simulink model "TLC"  (R2022b)
settings: configuration reference "ERT" (kept outside this file)
undefined symbols (not defined in the file): EGM, FID, IdcMin_P, kiIdcMax_P, kiIdcMin_P, kpIdcMax_P, kpIdcMin_P, OmMechnLimMin_P, pwrIdcMaxDev_P, pwrIdcMinDev_P, SC_fLoLim_C, SC_fUpLim_C, SC_PwrMax_P, SC_TrqMax_P, TQL, trqAddMax_P, trqAddMin_P, Ts_10ms
libraries: simulink x50, MathLib x8, DSMLib x2, slpidlib x1
(part 1 of 2)
settings Model: Creator=M00039784  LastModifiedBy=M00039784
settings ConfigSetRef: SourceName=ERT  SourceLocation=Base Workspace

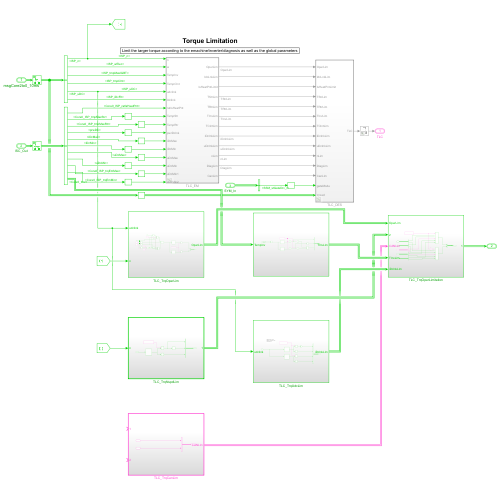
[thumbnail: Simulink's stored preview of the top-level diagram]
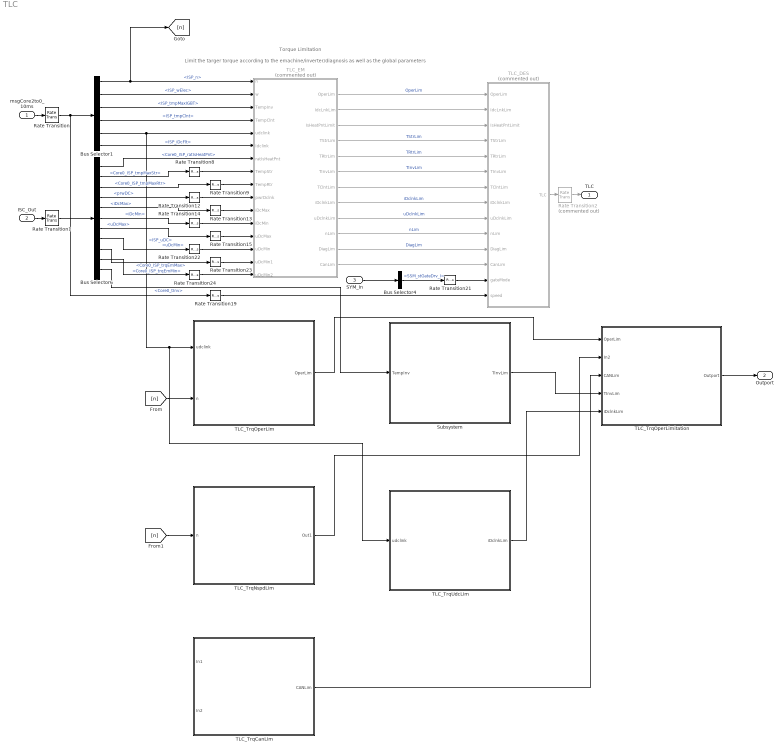
== system TLC ==
  note: Torque Limitation
  note: Limit the targer torque according to the emachine/inverter/diagnosis as well as the global parameters
  msgCore2to0_10ms : Inport  OutDataTypeStr=Bus: Sig10ms20ST
  ISC_Out : Inport  Port=2  OutDataTypeStr=Bus: Core0_ISP_Out
  SYM_In : Inport  Port=3  OutDataTypeStr=Bus: Core0_SSM_Out
  Bus Selector1 : BusSelector  OutputSignals=ISP_n,ISP_wElec,ISP_tmpMaxIGBT,ISP_tmpClnt,ISP_uDC,ISP_iDcFlt
  Bus Selector4 : BusSelector  OutputSignals=SSM_stGateDrv_I
  Bus Selector6 : BusSelector  OutputSignals=Core0_ISP_tmpOut.Core0_ISP_ratIsHeatPnt,Core0_ISP_tmpOut.Core0_ISP_tmpMaxStr,Core0_ISP_tmpOut.Core0_ISP_tmpMaxRtr,Core0_ISP_ComCmd.Core0_ISP_Dcx.prwDC,Core0_ISP_ComCmd.Core0_ISP_Dcx.iDcMax,Core0_ISP_ComCmd.Core0_ISP_Dcx.iDcMin,Core0_ISP_ComCmd.Core0_ISP_Dcx.uDcMax,Core0_ISP_ComCmd.Core0_ISP_Dcx.uDcMin,Core0_ISP_ComCmd.Core0_ISP_trqx.Core0_ISP_trqEmMax,Core0_ISP_ComCmd.Core0_ISP_trqx.Core0_ISP_trqEmMin,Core0_ISP_AnaOut.Core0_ISP_tInvx.Core0_tInv
  Rate Transition : RateTransition  OutPortSampleTime=Ts_10ms
  Rate Transition1 : RateTransition  OutPortSampleTime=Ts_10ms
  Rate Transition{8..9,12..15,19,22..24} (10 alike) : RateTransition
  Rate Transition2 : RateTransition  Commented=on  OutPortSampleTime=Ts_10ms
  Rate Transition21 : RateTransition  InitialCondition=EGM.Shortcircuit
  Subsystem : Subsystem
  TLC_DES : Subsystem  Commented=on  TreatAsAtomicUnit=on  SystemSampleTime=Ts_10ms
  TLC_EM : Subsystem  Commented=on  TreatAsAtomicUnit=on  SystemSampleTime=Ts_10ms
  TLC_TrqCanLim : Subsystem  TreatAsAtomicUnit=on
  TLC_TrqNspdLim : Subsystem  TreatAsAtomicUnit=on
  TLC_TrqOperLim : Subsystem
  TLC_TrqOperLimitation : Subsystem
  TLC_TrqUdcLim : Subsystem
  TLC : Outport  OutDataTypeStr=Bus: Core0_TLC_Out  VectorParamsAs1DForOutWhenUnconnected=off
  Outport : Outport  Port=2  OutDataTypeStr=Bus: Core0_TLC_TrqOut
  wires:
  TLC_EM/3(IsHeatPntLimit) -> TLC_DES/3(IsHeatPntLimit)
  Bus Selector6/1 -> TLC_EM/7(ratIsHeatPnt)  "<Core0_ISP_ratIsHeatPnt>"
  Bus Selector1/6 -> TLC_EM/6(Idclink)  "<ISP_iDcFlt>"
  TLC_EM/2(IdcLnkLim) -> TLC_DES/2(IdcLnkLim)
  Bus Selector1/5 -> TLC_TrqUdcLim/1(udclink), TLC_TrqOperLim/1(udclink), TLC_EM/5(udclink)  "<ISP_uDC>"
  Bus Selector6/10 -> Rate Transition24/1  "<Core0_ISP_trqEmMin>"
  Bus Selector1/3 -> TLC_EM/3(TempInv)  "<ISP_tmpMaxIGBT>"
  Bus Selector1/2 -> TLC_EM/2(w)  "<ISP_wElec>"
  SYM_In/1 -> Bus Selector4/1
  Bus Selector6/8 -> Rate Transition22/1  "<uDcMin>"
  TLC_EM/7(TClntLim) -> TLC_DES/7(TClntLim)
  Rate Transition19/1 -> TLC_DES/14(speed)
  Rate Transition24/1 -> TLC_EM/16(uDcMin2)
  Bus Selector6/7 -> Rate Transition15/1  "<uDcMax>"
  Bus Selector1/4 -> TLC_EM/4(TempClnt)  "<ISP_tmpClnt>"
  Bus Selector4/1 -> Rate Transition21/1  "<SSM_stGateDrv_I>"
  Bus Selector6/2 -> Rate Transition8/1  "<Core0_ISP_tmpMaxStr>"
  Rate Transition23/1 -> TLC_EM/15(uDcMin1)
  TLC_EM/8(iDclnkLim) -> TLC_DES/8(iDclnkLim)  "iDclnkLim"
  Rate Transition22/1 -> TLC_EM/14(uDcMin)
  Rate Transition12/1 -> TLC_EM/10(pwrDclnk)
  Rate Transition8/1 -> TLC_EM/8(TempStr)
  TLC_DES/1(TLC) -> Rate Transition2/1
  Rate Transition15/1 -> TLC_EM/13(uDcMax)
  Bus Selector6/4 -> Rate Transition12/1  "<prwDC>"
  Rate Transition14/1 -> TLC_EM/12(iDcMin)
  msgCore2to0_10ms/1 -> Rate Transition/1
  TLC_EM/5(TRtrLim) -> TLC_DES/5(TRtrLim)  "TRtrLim"
  Bus Selector6/3 -> Rate Transition9/1  "<Core0_ISP_tmpMaxRtr>"
  Bus Selector6/5 -> Rate Transition13/1  "<iDcMax>"
  TLC_EM/6(TInvLim) -> TLC_DES/6(TInvLim)  "TInvLim"
  ISC_Out/1 -> Rate Transition1/1
  TLC_EM/10(nLim) -> TLC_DES/10(nLim)  "nLim"
  TLC_EM/11(DiagLim) -> TLC_DES/11(DiagLim)  "DiagLim"
  Bus Selector1/1 -> [n], TLC_EM/1(n)  "<ISP_n>"
  TLC_EM/4(TStrLim) -> TLC_DES/4(TStrLim)  "TStrLim"
  TLC_EM/1(OperLim) -> TLC_DES/1(OperLim)  "OperLim"
  Bus Selector6/6 -> Rate Transition14/1  "<iDcMin>"
  TLC_EM/9(uDclnkLim) -> TLC_DES/9(uDclnkLim)  "uDclnkLim"
  Rate Transition21/1 -> TLC_DES/13(gateMode)
  Bus Selector6/9 -> Rate Transition23/1  "<Core0_ISP_trqEmMax>"
  TLC_EM/12(CanLim) -> TLC_DES/12(CanLim)
  Rate Transition9/1 -> TLC_EM/9(TempRtr)
  Rate Transition13/1 -> TLC_EM/11(iDcMax)
  Rate Transition/1 -> Rate Transition19/1, Bus Selector1/1
  Rate Transition1/1 -> Bus Selector6/1
  Rate Transition2/1 -> TLC/1
  [n] -> TLC_TrqOperLim/2(n)
  [n] -> TLC_TrqNspdLim/1(n)
  TLC_TrqOperLim/1(OperLim) -> TLC_TrqOperLimitation/1(OperLim)
  TLC_TrqNspdLim/1(Out1) -> TLC_TrqOperLimitation/2(In2)
  TLC_TrqCanLim/1(CANLim) -> TLC_TrqOperLimitation/3(CANLim)
  Subsystem/1(TInvLim) -> TLC_TrqOperLimitation/4(TInvLim)
  TLC_TrqUdcLim/1(iDclnkLim) -> TLC_TrqOperLimitation/5(iDclnkLim)
  TLC_TrqOperLimitation/1(Outport) -> Outport/1
  Bus Selector6/11 -> Subsystem/1(TempInv)  "<Core0_tInv>"

== system TLC/Subsystem ==
  TempInv : Inport
  Bus Creator : BusCreator  Inputs=3
  Bus Selector : BusSelector  OutputSignals=Core0_ISP_IGBTTemp1,Core0_ISP_IGBTTemp2
  GLB_TrqMax_P2 : Constant  Value=SC_TrqMax_P  OutDataTypeStr=single
  Logical Operator : Logic  Operator=OR  AllPortsSameDT=off  OutDataTypeStr=boolean
  Max : MinMax  Function=max  Inputs=2
  Product : Product
  Product1 : Product
  Relational Operator : RelationalOperator  OutDataTypeStr=boolean  RndMeth=Simplest  InputSameDT=off
  Relational Operator1 : RelationalOperator  OutDataTypeStr=boolean  RndMeth=Simplest  InputSameDT=off
  Unary Minus : UnaryMinus
  trqGenTInvLim_T : Lookup_n-D  NumberOfTableDimensions=1  DataSpecification=Lookup table object  LookupTableObject=trqGenTInvLim_T  BreakpointsForDimension1=[100 125 135]  BeginIndexSearchUsingPreviousIndexResult=on  Table=[1 0.8 0]  ExtrapMethod=Clip  UseLastTableValue=on  InternalRulePriority=Speed  OutDataTypeStr=Inherit: Inherit from 'Table data'  RndMeth=Simplest
  trqMotTInvLim_T : Lookup_n-D  NumberOfTableDimensions=1  DataSpecification=Lookup table object  LookupTableObject=trqMotTInvLim_T  BreakpointsForDimension1=[100 125 135]  BeginIndexSearchUsingPreviousIndexResult=on  Table=[1 0.8 0]  ExtrapMethod=Clip  UseLastTableValue=on  InternalRulePriority=Speed  OutDataTypeStr=Inherit: Inherit from 'Table data'  RndMeth=Simplest
  TInvLim : Outport  VectorParamsAs1DForOutWhenUnconnected=off
  wires:
  Logical Operator/1 -> Bus Creator/3  "bTrqTinvLimActv"
  trqGenTInvLim_T/1 -> Product1/2
  Relational Operator1/1 -> Logical Operator/2  "bTrqGenTInvLimActv"
  Bus Creator/1 -> TInvLim/1
  Relational Operator/1 -> Logical Operator/1  "bTrqMotTInvLimActv"
  GLB_TrqMax_P2/1 -> Relational Operator1/1, Relational Operator/1, Product1/1, Product/1
  trqMotTInvLim_T/1 -> Product/2
  Product1/1 -> Unary Minus/1, Relational Operator1/2
  Unary Minus/1 -> Bus Creator/2  "trqGenTInvLim"
  Max/1 -> trqGenTInvLim_T/1, trqMotTInvLim_T/1
  Product/1 -> Bus Creator/1, Relational Operator/2  "trqMotTInvLim"
  TempInv/1 -> Bus Selector/1
  Bus Selector/1 -> Max/1  "<Core0_ISP_IGBTTemp1>"
  Bus Selector/2 -> Max/2  "<Core0_ISP_IGBTTemp2>"

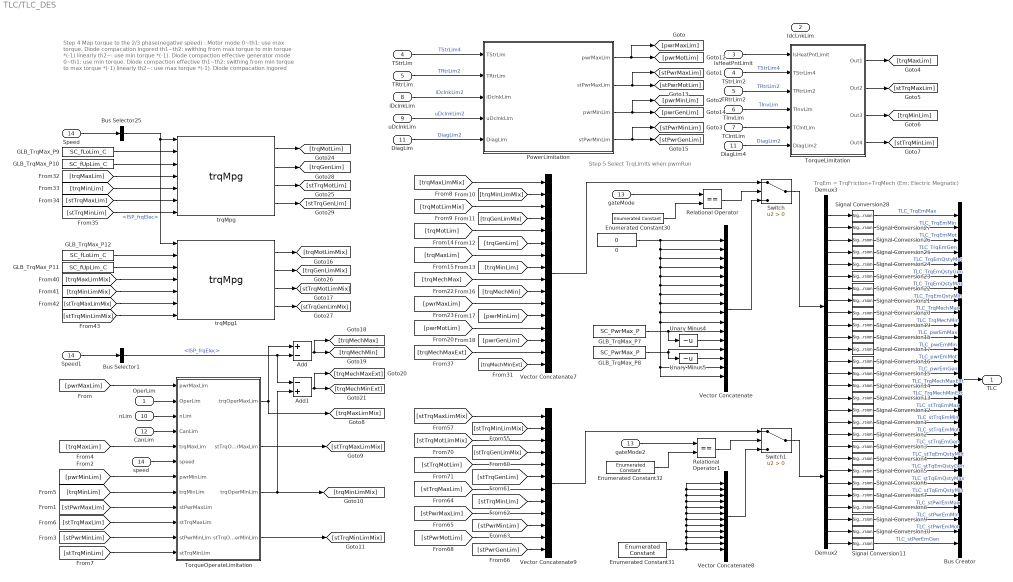
== system TLC/TLC_DES ==
  note: Step 4 Map torque to the 2/3 phase(negative speed) :
      | Motor mode
      | 0~th1: use max torque. Diode compacation ingored
      | th1~th2: swithing from max torque to min torque *(-1) linearly
      | th2~: use min torque *(-1). Diode compaction effective
      | generator mode
      | 0~th1: use min torque. Diode compaction effective
      | th1~th2: swithing from min torque to max torque *(-1) linearly
      | th2~: use max torque *(-1). Diode compacation ingored
  note: TrqEm = TrqFriction+TrqMech (Em: Electric Megnatic)
  note: Step 5 Select TrqLimits when pwmRun
  OperLim : Inport
  IdcLnkLim : Inport  Port=2
  IsHeatPntLimit : Inport  Port=3
  TStrLim : Inport  Port=4
  TRtrLim : Inport  Port=5
  TInvLim : Inport  Port=6
  TClntLim : Inport  Port=7
  iDclnkLim : Inport  Port=8
  uDclnkLim : Inport  Port=9
  nLim : Inport  Port=10
  DiagLim : Inport  Port=11
  CanLim : Inport  Port=12
  gateMode : Inport  Port=13
  speed : Inport  Port=14
  0 : Constant  Value=0  OutDataTypeStr=single
  Add : Sum  Inputs=+-
  Add1 : Sum  Inputs=-+
  Bus Creator : BusCreator  Inputs=28
  Bus Selector1 : BusSelector  OutputSignals=ISP_frqElec
  Bus Selector25 : BusSelector  OutputSignals=ISP_frqElec
  Demux2 : Demux  Outputs=12
  Demux3 : Demux  Outputs=16
  DiagLim4 : InportShadow  Port=11
  Enumerated Constant30 : simulink/Sources/Enumerated Constant  OutDataTypeStr=Enum: EGM  Value=EGM.PWMRun  SampleTime=inf
  Enumerated Constant31 : simulink/Sources/Enumerated Constant  OutDataTypeStr=Enum: TQL  Value=TQL.Inactive  SampleTime=inf
  Enumerated Constant32 : simulink/Sources/Enumerated Constant  OutDataTypeStr=Enum: EGM  Value=EGM.PWMRun  SampleTime=inf
  GLB_TrqMax_P10 : Constant  Value=SC_fUpLim_C  OutDataTypeStr=single
  GLB_TrqMax_P11 : Constant  Value=SC_fUpLim_C  OutDataTypeStr=single
  GLB_TrqMax_P12 : Constant  Value=SC_fLoLim_C  OutDataTypeStr=single
  GLB_TrqMax_P7 : Constant  Value=SC_PwrMax_P  OutDataTypeStr=single
  GLB_TrqMax_P8 : Constant  Value=SC_PwrMax_P  OutDataTypeStr=single
  GLB_TrqMax_P9 : Constant  Value=SC_fLoLim_C  OutDataTypeStr=single
  PowerLimitation : Subsystem
  Relational Operator : RelationalOperator  Operator===  OutDataTypeStr=boolean  RndMeth=Simplest  InputSameDT=off
  Relational Operator1 : RelationalOperator  Operator===  OutDataTypeStr=boolean  RndMeth=Simplest  InputSameDT=off
  Signal Conversion{1..28} (28 alike) : SignalConversion  OverrideOpt=off
  Speed : InportShadow  Port=14
  Speed1 : InportShadow  Port=14
  Switch : Switch  Criteria=u2 > Threshold  SaturateOnIntegerOverflow=off  InputSameDT=off
  Switch1 : Switch  Criteria=u2 > Threshold  SaturateOnIntegerOverflow=off  InputSameDT=off
  TRtrLim2 : InportShadow  Port=5
  TStrLim2 : InportShadow  Port=4
  TorqueLimitation : Subsystem
  TorqueOperateLimitation : Subsystem
  Unary Minus4 : UnaryMinus
  Unary Minus5 : UnaryMinus
  Vector Concatenate : Concatenate  NumInputs=16
  Vector Concatenate7 : Concatenate  NumInputs=16
  Vector Concatenate8 : Concatenate  NumInputs=12
  Vector Concatenate9 : Concatenate  NumInputs=12
  gateMode2 : InportShadow  Port=13
  trqMpg : MathLib/trqMpg  SystemSampleTime=-1  VariantActivationTime=update diagram  Latency=0  AutoFrameSizeCalculation=off
  trqMpg1 : MathLib/trqMpg  SystemSampleTime=-1  VariantActivationTime=update diagram  Latency=0  AutoFrameSizeCalculation=off
  TLC : Outport  VectorParamsAs1DForOutWhenUnconnected=off
  wires:
  Speed/1 -> Bus Selector25/1
  trqMpg/1 -> [trqMotLim]
  trqMpg/3 -> [stTrqMotLim]
  trqMpg/2 -> [trqGenLim]
  trqMpg/4 -> [stTrqGenLim]
  Bus Selector25/1 -> trqMpg1/1, trqMpg/1  "<ISP_frqElec>"
  trqMpg1/1 -> [trqMotLimMix]
  trqMpg1/3 -> [stTrqMotLimMix]
  trqMpg1/2 -> [trqGenLimMix]
  trqMpg1/4 -> [stTrqGenLimMix]
  TorqueOperateLimitation/1(trqOperMaxLim) -> [trqMaxLimMix], Add/1
  TorqueOperateLimitation/3(trqOperMinLim) -> Add1/2, [trqMinLimMix]
  Bus Selector1/1 -> Add1/1, Add/2  "<ISP_frqElec>"
  Add/1 -> [trqMechMax], [trqMechMin]
  Add1/1 -> [trqMechMaxExt], [trqMechMinExt]
  [stTrqMinLim] -> trqMpg/7
  [stTrqMaxLim] -> trqMpg/6
  [trqMinLim] -> trqMpg/5
  [trqMaxLim] -> trqMpg/4
  GLB_TrqMax_P9/1 -> trqMpg/2
  GLB_TrqMax_P10/1 -> trqMpg/3
  [stTrqMinLimMix] -> trqMpg1/7
  [stTrqMaxLimMix] -> trqMpg1/6
  [trqMinLimMix] -> trqMpg1/5
  [trqMaxLimMix] -> trqMpg1/4
  GLB_TrqMax_P12/1 -> trqMpg1/2
  GLB_TrqMax_P11/1 -> trqMpg1/3
  PowerLimitation/1(pwrMaxLim) -> [pwrMaxLim], [pwrMotLim]
  PowerLimitation/2(stPwrMaxLim) -> [stPwrMaxLim], [stPwrMotLim]
  PowerLimitation/3(pwrMinLim) -> [pwrMinLim], [pwrGenLim]
  PowerLimitation/4(stPwrMinLim) -> [stPwrMinLim], [stPwrGenLim]
  TStrLim/1 -> PowerLimitation/1(TStrLim)  "TStrLim4"
  TRtrLim/1 -> PowerLimitation/2(TRtrLim)  "TRtrLim2"
  iDclnkLim/1 -> PowerLimitation/3(iDclnkLim)  "iDclnkLim2"
  uDclnkLim/1 -> PowerLimitation/4(uDclnkLim)  "uDclnkLim2"
  DiagLim/1 -> PowerLimitation/5(DiagLim)  "DiagLim2"
  TStrLim2/1 -> TorqueLimitation/2(TStrLim4)  "TStrLim4"
  TRtrLim2/1 -> TorqueLimitation/3(TRtrLim2)  "TRtrLim2"
  TInvLim/1 -> TorqueLimitation/4(TInvLim)  "TInvLim"
  DiagLim4/1 -> TorqueLimitation/6(DiagLim2)  "DiagLim2"
  TorqueLimitation/1(Out1) -> [trqMaxLim]
  TorqueLimitation/2(Out2) -> [stTrqMaxLim]
  TorqueLimitation/3(Out3) -> [trqMinLim]
  TorqueLimitation/4(Out4) -> [stTrqMinLim]
  [pwrMaxLim] -> TorqueOperateLimitation/1(pwrMaxLim)
  OperLim/1 -> TorqueOperateLimitation/2(OperLim)
  nLim/1 -> TorqueOperateLimitation/3(nLim)
  CanLim/1 -> TorqueOperateLimitation/4(CanLim)
  [trqMaxLim] -> TorqueOperateLimitation/5(trqMaxLim)
  speed/1 -> TorqueOperateLimitation/6(speed)
  [pwrMinLim] -> TorqueOperateLimitation/7(pwrMinLim)
  [trqMinLim] -> TorqueOperateLimitation/8(trqMinLim)
  TorqueOperateLimitation/2(stTrqOperMaxLim) -> [stTrqMaxLimMix]
  TorqueOperateLimitation/4(stTrqOperMinLim) -> [stTrqMinLimMix]
  [stPwrMaxLim] -> TorqueOperateLimitation/9(stPwrMaxLim)
  [stTrqMaxLim] -> TorqueOperateLimitation/10(stTrqMaxLim)
  [stTrqMinLim] -> TorqueOperateLimitation/12(stTrqMinLim)
  [stPwrMinLim] -> TorqueOperateLimitation/11(stPwrMinLim)
  Enumerated Constant30/1 -> Relational Operator/2
  Relational Operator/1 -> Switch/2
  0/1 -> Vector Concatenate/2, Vector Concatenate/3, Vector Concatenate/4, Vector Concatenate/5, Vector Concatenate/6, Vector Concatenate/7, Vector Concatenate/8, Vector Concatenate/9, Vector Concatenate/10, Vector Concatenate/16, Vector Concatenate/15, Vector Concatenate/1
  GLB_TrqMax_P7/1 -> Vector Concatenate/11, Unary Minus4/1
  GLB_TrqMax_P8/1 -> Vector Concatenate/13, Unary Minus5/1
  Demux3/7 -> Signal Conversion22/1
  Demux3/6 -> Signal Conversion23/1
  Demux3/8 -> Signal Conversion21/1
  Demux3/5 -> Signal Conversion24/1
  Demux3/9 -> Signal Conversion20/1
  Demux3/4 -> Signal Conversion25/1
  Demux3/3 -> Signal Conversion26/1
  Demux3/10 -> Signal Conversion19/1
  Demux3/2 -> Signal Conversion27/1
  Demux3/11 -> Signal Conversion18/1
  Demux3/1 -> Signal Conversion28/1
  Demux3/12 -> Signal Conversion17/1
  Demux3/13 -> Signal Conversion16/1
  Demux3/14 -> Signal Conversion15/1
  Demux2/1 -> Signal Conversion12/1
  Demux2/2 -> Signal Conversion1/1
  Demux2/3 -> Signal Conversion2/1
  Demux2/4 -> Signal Conversion3/1
  Demux2/5 -> Signal Conversion4/1
  Demux2/6 -> Signal Conversion5/1
  Demux2/7 -> Signal Conversion6/1
  Demux2/8 -> Signal Conversion7/1
  Demux2/9 -> Signal Conversion8/1
  Demux2/10 -> Signal Conversion9/1
  Demux2/11 -> Signal Conversion10/1
  Demux2/12 -> Signal Conversion11/1
  Demux3/15 -> Signal Conversion14/1
  Demux3/16 -> Signal Conversion13/1
  [trqMotLimMix] -> Vector Concatenate7/3
  [trqMaxLimMix] -> Vector Concatenate7/1
  [trqMinLimMix] -> Vector Concatenate7/2
  Vector Concatenate7/1 -> Switch/1
  Vector Concatenate/1 -> Switch/3
  Switch/1 -> Demux3/1
  [trqGenLimMix] -> Vector Concatenate7/4
  [trqMaxLim] -> Vector Concatenate7/7
  [trqMotLim] -> Vector Concatenate7/5
  [trqGenLim] -> Vector Concatenate7/6
  [trqMinLim] -> Vector Concatenate7/8
  [pwrMaxLim] -> Vector Concatenate7/11
  [trqMechMax] -> Vector Concatenate7/9
  [pwrMotLim] -> Vector Concatenate7/13
  [trqMechMaxExt] -> Vector Concatenate7/15
  [trqMechMinExt] -> Vector Concatenate7/16
  [pwrGenLim] -> Vector Concatenate7/14
  [trqMechMin] -> Vector Concatenate7/10
  [pwrMinLim] -> Vector Concatenate7/12
  Bus Creator/1 -> TLC/1
  Unary Minus5/1 -> Vector Concatenate/14
  Unary Minus4/1 -> Vector Concatenate/12
  Enumerated Constant31/1 -> Vector Concatenate8/1, Vector Concatenate8/2, Vector Concatenate8/3, Vector Concatenate8/4, Vector Concatenate8/5, Vector Concatenate8/6, Vector Concatenate8/7, Vector Concatenate8/8, Vector Concatenate8/9, Vector Concatenate8/10, Vector Concatenate8/11, Vector Concatenate8/12
  Vector Concatenate9/1 -> Switch1/1
  [stPwrGenLim] -> Vector Concatenate9/12
  [stPwrMinLim] -> Vector Concatenate9/10
  [stTrqMinLim] -> Vector Concatenate9/8
  [stTrqGenLim] -> Vector Concatenate9/6
  [stTrqGenLimMix] -> Vector Concatenate9/4
  [stPwrMotLim] -> Vector Concatenate9/11
  [stTrqMinLimMix] -> Vector Concatenate9/2
  [stPwrMaxLim] -> Vector Concatenate9/9
  [stTrqMaxLim] -> Vector Concatenate9/7
  [stTrqMotLim] -> Vector Concatenate9/5
  [stTrqMotLimMix] -> Vector Concatenate9/3
  [stTrqMaxLimMix] -> Vector Concatenate9/1
  Enumerated Constant32/1 -> Relational Operator1/2
  Relational Operator1/1 -> Switch1/2
  Vector Concatenate8/1 -> Switch1/3
  Switch1/1 -> Demux2/1
  Signal Conversion1/1 -> Bus Creator/18  "TLC_stTrqEmMin"
  Signal Conversion2/1 -> Bus Creator/19  "TLC_stTrqEmMot"
  Signal Conversion3/1 -> Bus Creator/20  "TLC_stTrqEmGen"
  Signal Conversion4/1 -> Bus Creator/21  "TLC_stTqEmQstyMot"
  Signal Conversion5/1 -> Bus Creator/22  "TLC_stTqEmQstyGen"
  Signal Conversion6/1 -> Bus Creator/23  "TLC_stTqEmQstyMax"
  Signal Conversion7/1 -> Bus Creator/24  "TLC_stTqEmQstyMin"
  Signal Conversion8/1 -> Bus Creator/25  "TLC_stPwrEmMax"
  Signal Conversion9/1 -> Bus Creator/26  "TLC_stPwrEmMin"
  Signal Conversion10/1 -> Bus Creator/27  "TLC_stPwrEmMot"
  Signal Conversion11/1 -> Bus Creator/28  "TLC_stPwrEmGen"
  Signal Conversion12/1 -> Bus Creator/17  "TLC_stTrqEmMax"
  Signal Conversion13/1 -> Bus Creator/16  "TLC_TrqMechMinExt"
  Signal Conversion14/1 -> Bus Creator/15  "TLC_TrqMechMaxExt"
  Signal Conversion15/1 -> Bus Creator/14  "TLC_pwrEmGen"
  Signal Conversion16/1 -> Bus Creator/13  "TLC_pwrEmMot"
  Signal Conversion17/1 -> Bus Creator/12  "TLC_pwrEmMin"
  Signal Conversion18/1 -> Bus Creator/11  "TLC_pwrEmMax"
  Signal Conversion19/1 -> Bus Creator/10  "TLC_TrqMechMin"
  Signal Conversion20/1 -> Bus Creator/9  "TLC_TrqMechMax"
  Signal Conversion21/1 -> Bus Creator/8  "TLC_TrqEmQstyMin"
  Signal Conversion22/1 -> Bus Creator/7  "TLC_TrqEmQstyMax"
  Signal Conversion23/1 -> Bus Creator/6  "TLC_TrqEmQstyGen"
  Signal Conversion24/1 -> Bus Creator/5  "TLC_TrqEmQstyMot"
  Signal Conversion25/1 -> Bus Creator/4  "TLC_TrqEmGen"
  Signal Conversion26/1 -> Bus Creator/3  "TLC_TrqEmMot"
  Signal Conversion27/1 -> Bus Creator/2  "TLC_TrqEmMin"
  Signal Conversion28/1 -> Bus Creator/1  "TLC_TrqEmMax"
  gateMode/1 -> Relational Operator/1
  gateMode2/1 -> Relational Operator1/1
  Speed1/1 -> Bus Selector1/1
  IsHeatPntLimit/1 -> TorqueLimitation/1(IsHeatPntLimit)
  TClntLim/1 -> TorqueLimitation/5(TClntLim)

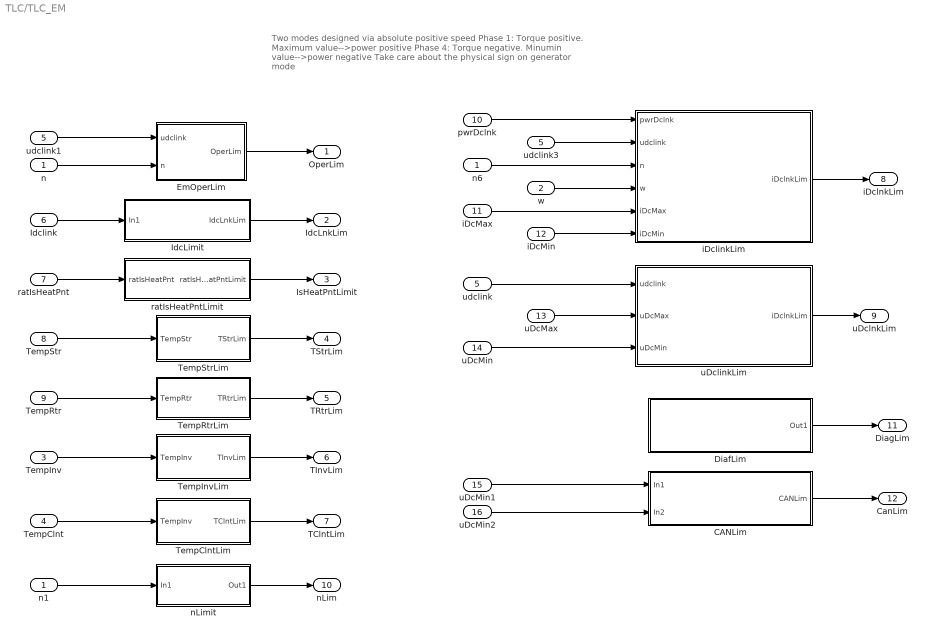
== system TLC/TLC_EM ==
  note: Two modes designed via absolute positive speed
      | Phase 1: Torque  positive. Maximum value-->power positive
      | Phase 4: Torque negative. Minumin value-->power negative
      | Take care about the physical sign on generator mode
  n : Inport
  w : Inport  Port=2
  TempInv : Inport  Port=3
  TempClnt : Inport  Port=4
  udclink : Inport  Port=5
  Idclink : Inport  Port=6
  ratIsHeatPnt : Inport  Port=7
  TempStr : Inport  Port=8
  TempRtr : Inport  Port=9
  pwrDclnk : Inport  Port=10
  iDcMax : Inport  Port=11
  iDcMin : Inport  Port=12
  uDcMax : Inport  Port=13
  uDcMin : Inport  Port=14
  uDcMin1 : Inport  Port=15
  uDcMin2 : Inport  Port=16
  CANLim : Subsystem  TreatAsAtomicUnit=on
  DiafLim : Subsystem  TreatAsAtomicUnit=on
  EmOperLim : Subsystem  TreatAsAtomicUnit=on
  IdcLimit : Subsystem  TreatAsAtomicUnit=on
  TempClntLim : Subsystem  TreatAsAtomicUnit=on
  TempInvLim : Subsystem  TreatAsAtomicUnit=on
  TempRtrLim : Subsystem  TreatAsAtomicUnit=on
  TempStrLim : Subsystem  TreatAsAtomicUnit=on
  iDclinkLim : Subsystem  TreatAsAtomicUnit=on
  n1 : InportShadow
  n6 : InportShadow
  nLimit : Subsystem  TreatAsAtomicUnit=on
  ratIsHeatPntLimit : Subsystem  TreatAsAtomicUnit=on
  uDclinkLim : Subsystem  TreatAsAtomicUnit=on
  udclink1 : InportShadow  Port=5
  udclink3 : InportShadow  Port=5
  OperLim : Outport  VectorParamsAs1DForOutWhenUnconnected=off
  IdcLnkLim : Outport  Port=2  VectorParamsAs1DForOutWhenUnconnected=off
  IsHeatPntLimit : Outport  Port=3  VectorParamsAs1DForOutWhenUnconnected=off
  TStrLim : Outport  Port=4  VectorParamsAs1DForOutWhenUnconnected=off
  TRtrLim : Outport  Port=5  VectorParamsAs1DForOutWhenUnconnected=off
  TInvLim : Outport  Port=6  VectorParamsAs1DForOutWhenUnconnected=off
  TClntLim : Outport  Port=7  VectorParamsAs1DForOutWhenUnconnected=off
  iDclnkLim : Outport  Port=8  VectorParamsAs1DForOutWhenUnconnected=off
  uDclnkLim : Outport  Port=9  VectorParamsAs1DForOutWhenUnconnected=off
  nLim : Outport  Port=10  VectorParamsAs1DForOutWhenUnconnected=off
  DiagLim : Outport  Port=11  VectorParamsAs1DForOutWhenUnconnected=off
  CanLim : Outport  Port=12  VectorParamsAs1DForOutWhenUnconnected=off
  wires:
  TempInvLim/1(TInvLim) -> TInvLim/1
  TempInv/1 -> TempInvLim/1(TempInv)
  udclink1/1 -> EmOperLim/1(udclink)
  n/1 -> EmOperLim/2(n)
  EmOperLim/1(OperLim) -> OperLim/1
  TempStr/1 -> TempStrLim/1(TempStr)
  TempStrLim/1(TStrLim) -> TStrLim/1
  TempRtr/1 -> TempRtrLim/1(TempRtr)
  TempRtrLim/1(TRtrLim) -> TRtrLim/1
  udclink3/1 -> iDclinkLim/2(udclink)
  n6/1 -> iDclinkLim/3(n)
  iDcMax/1 -> iDclinkLim/5(iDcMax)
  pwrDclnk/1 -> iDclinkLim/1(pwrDclnk)
  w/1 -> iDclinkLim/4(w)
  iDcMin/1 -> iDclinkLim/6(iDcMin)
  iDclinkLim/1(iDclnkLim) -> iDclnkLim/1
  udclink/1 -> uDclinkLim/1(udclink)
  uDcMax/1 -> uDclinkLim/2(uDcMax)
  uDcMin/1 -> uDclinkLim/3(uDcMin)
  uDclinkLim/1(iDclnkLim) -> uDclnkLim/1
  n1/1 -> nLimit/1(In1)
  nLimit/1(Out1) -> nLim/1
  DiafLim/1(Out1) -> DiagLim/1
  CANLim/1(CANLim) -> CanLim/1
  uDcMin1/1 -> CANLim/1(In1)
  uDcMin2/1 -> CANLim/2(In2)
  Idclink/1 -> IdcLimit/1(In1)
  IdcLimit/1(IdcLnkLim) -> IdcLnkLim/1
  ratIsHeatPnt/1 -> ratIsHeatPntLimit/1(ratIsHeatPnt)
  ratIsHeatPntLimit/1(ratIsHeatPntLimit) -> IsHeatPntLimit/1
  TempClnt/1 -> TempClntLim/1(TempInv)
  TempClntLim/1(TClntLim) -> TClntLim/1

== system TLC/TLC_TrqCanLim ==
  In1 : Inport
  In2 : Inport  Port=2
  Bus Creator : BusCreator  Inputs=2
  CANLim : Outport  VectorParamsAs1DForOutWhenUnconnected=off
  wires:
  In1/1 -> Bus Creator/1  "trqMotCanLim"
  In2/1 -> Bus Creator/2  "trqGenCanLim"
  Bus Creator/1 -> CANLim/1

== system TLC/TLC_TrqNspdLim ==
  n : Inport
  Bus Creator : BusCreator  Inputs=3
  Compare To Constant : simulink/Logic and Bit Operations/Compare To Constant  relop=<  const=1  OutDataTypeStr=boolean
  GLB_PwrMax_P : Constant  Value=SC_TrqMax_P  OutDataTypeStr=single
  Product : Product
  Unary Minus3 : UnaryMinus
  pwrGenMotnLim_T : Lookup_n-D  NumberOfTableDimensions=1  DataSpecification=Lookup table object  LookupTableObject=pwrGenMotnLim_T  BreakpointsForDimension1=[-3500 -3000 0 7000 7200]  BeginIndexSearchUsingPreviousIndexResult=on  Table=[0 1 1 1 0]  ExtrapMethod=Clip  UseLastTableValue=on  InternalRulePriority=Speed  OutDataTypeStr=Inherit: Inherit from 'Table data'  RndMeth=Simplest
  Out1 : Outport  VectorParamsAs1DForOutWhenUnconnected=off
  wires:
  pwrGenMotnLim_T/1 -> Compare To Constant/1, Product/2
  GLB_PwrMax_P/1 -> Product/1
  Compare To Constant/1 -> Bus Creator/3  "bTrqnLimActv"
  Unary Minus3/1 -> Bus Creator/2  "trqGennLim"
  Bus Creator/1 -> Out1/1
  n/1 -> pwrGenMotnLim_T/1
  Product/1 -> Bus Creator/1, Unary Minus3/1  "trqMotnLim"

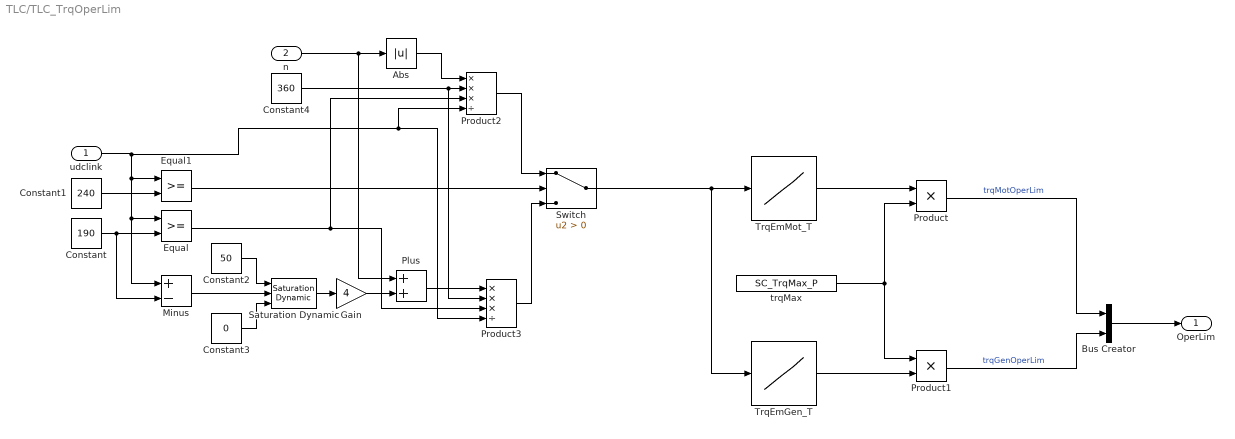
== system TLC/TLC_TrqOperLim ==
  udclink : Inport
  n : Inport  Port=2
  Abs : Abs  SaturateOnIntegerOverflow=off
  Bus Creator : BusCreator  Inputs=2
  Constant : Constant  Value=190  OutDataTypeStr=single
  Constant1 : Constant  Value=240  OutDataTypeStr=single
  Constant2 : Constant  Value=50  OutDataTypeStr=single
  Constant3 : Constant  Value=0  OutDataTypeStr=single
  Constant4 : Constant  Value=360  OutDataTypeStr=single
  Equal : RelationalOperator  OutDataTypeStr=boolean  RndMeth=Simplest  InputSameDT=off
  Equal1 : RelationalOperator  OutDataTypeStr=boolean  RndMeth=Simplest  InputSameDT=off
  Gain : Gain  Gain=4
  Minus : Sum  Inputs=+-
  Plus : Sum
  Product : Product
  Product1 : Product
  Product2 : Product  Inputs=***/
  Product3 : Product  Inputs=***/
  Saturation Dynamic : simulink/Discontinuities/Saturation Dynamic  OutMin=[]  OutMax=[]  OutDataTypeStr=Inherit: Same as second input  OutDataType=fixdt(1, 16)  OutScaling=2^-10  DoSatur=off
  Switch : Switch  Criteria=u2 > Threshold  SaturateOnIntegerOverflow=off  InputSameDT=off
  TrqEmGen_T : Lookup_n-D  NumberOfTableDimensions=1  DataSpecification=Lookup table object  LookupTableObject=TrqEmGen_T  BreakpointsForDimension1=[250,300,350,400]  BreakpointsForDimension2=[0,500,1000,1500,2000,2500,3000,3500,4000,4500,5000,5500,6000,6500,7000,7500,8000,8500,9000,9500,10000,10500,11000,11500,12000,12500,13000,13500,14000,14500,15000]  BeginIndexSearchUsingPreviousIndexResult=on  Table=reshape([350,350,350,350,350,350,350,350,350,350,350,350,350,350,350,350,350,350,350,350,350,350,350,350,350,350,350,350,350,350,350,350,350,350,350,350,350,350,350,350,350,350,350,350,350,350,350,350,350,350,350,350,350,350,350,350,350,350,350,350,350,350,350,350,350,350,350,350,350,350,350,350,350,350,350,350,350,350,350,350,350,350,350,350,350,350,350,350,350,350,350,350,350,350,350,350,350,350,350,350,350,350,350,350,350,350,350,350,350,350,350,350,350,350,350,350,350,350,350,350,0,0,0,0],4,31)  ExtrapMethod=Clip  UseLastTableValue=on  InternalRulePriority=Speed  OutDataTypeStr=Inherit: Inherit from 'Table data'  RndMeth=Simplest
  TrqEmMot_T : Lookup_n-D  NumberOfTableDimensions=1  DataSpecification=Lookup table object  LookupTableObject=TrqEmMot_T  BreakpointsForDimension1=[0,500,1000,1500,2000,2500,3000,3500,4000,4500,5000,5500,6000,6500,7000,7500,8000,8500,9000,9500,10000,10500,11000,11500,12000,12500,13000,13500,14000,14500,15000]  BreakpointsForDimension2=[0,500,1000,1500,2000,2500,3000,3500,4000,4500,5000,5500,6000,6500,7000,7500,8000,8500,9000,9500,10000,10500,11000,11500,12000,12500,13000,13500,14000,14500,15000]  BeginIndexSearchUsingPreviousIndexResult=on  Table=[350,350,350,350,350,350,350,350,350,350,350,350,350,350,350,350,350,350,350,350,350,350,350,350,350,350,350,350,350,350,350,350,350,350,350,350,350,350,350,350,350,350,350,350,350,350,350,350,350,350,350,350,350,350,350,350,350,350,350,350,350,350,350,350,350,350,350,350,350,350,350,350,350,350,350,350,350,350,350,350,350,350,350,350,350,350,350,350,350,350,350,350,350,350,350,350,350,350,350,350,350,350,350,350,350,350,350,350,350,350,350,350,350,350,350,350,350,350,350,350,0,0,0,0]  ExtrapMethod=Clip  UseLastTableValue=on  InternalRulePriority=Speed  OutDataTypeStr=Inherit: Inherit from 'Table data'  RndMeth=Simplest
  trqMax : Constant  Value=SC_TrqMax_P  OutDataTypeStr=single
  OperLim : Outport  VectorParamsAs1DForOutWhenUnconnected=off
  wires:
  n/1 -> Abs/1, Plus/1
  Product1/1 -> Bus Creator/2  "trqGenOperLim"
  Product/1 -> Bus Creator/1  "trqMotOperLim"
  Bus Creator/1 -> OperLim/1
  TrqEmMot_T/1 -> Product/1
  Switch/1 -> TrqEmGen_T/1, TrqEmMot_T/1
  TrqEmGen_T/1 -> Product1/2
  trqMax/1 -> Product1/1, Product/2
  Constant/1 -> Minus/2, Equal/2
  Constant1/1 -> Equal1/2
  Equal1/1 -> Switch/2
  Minus/1 -> Saturation Dynamic/2
  Constant2/1 -> Saturation Dynamic/1
  Constant3/1 -> Saturation Dynamic/3
  Saturation Dynamic/1 -> Gain/1
  Abs/1 -> Product2/1
  Constant4/1 -> Product3/2, Product2/2
  Product2/1 -> Switch/1
  Gain/1 -> Plus/2
  Plus/1 -> Product3/1
  Product3/1 -> Switch/3
  udclink/1 -> Product3/4, Product2/4, Equal1/1, Minus/1, Equal/1
  Equal/1 -> Product3/3, Product2/3

== system TLC/TLC_TrqOperLimitation ==
  OperLim : Inport
  In2 : Inport  Port=2
  CANLim : Inport  Port=3
  TInvLim : Inport  Port=4
  iDclnkLim : Inport  Port=5
  Bus Creator : BusCreator  Inputs=2  OutDataTypeStr=Bus: Core0_TLC_TrqOut  NonVirtualBus=on
  Bus Selector : BusSelector  OutputSignals=trqMotOperLim,trqGenOperLim
  Bus Selector1 : BusSelector  OutputSignals=trqMotnLim,trqGennLim
  Bus Selector2 : BusSelector  OutputSignals=trqMotCanLim,trqGenCanLim
  Bus Selector3 : BusSelector  OutputSignals=trqMotTInvLim,trqGenTInvLim
  Bus Selector4 : BusSelector  OutputSignals=pwrMotUdclnkLim,signal1
  GLB_TrqMax_P2 : Constant  Value=SC_TrqMax_P  OutDataTypeStr=single
  Gain : Gain  Gain=-1
  Max : MinMax  Function=max  Inputs=6
  Min : MinMax  Inputs=6
  Outport : Outport  OutDataTypeStr=Bus: Core0_TLC_TrqOut
  wires:
  OperLim/1 -> Bus Selector/1
  GLB_TrqMax_P2/1 -> Min/1, Gain/1
  Bus Selector/1 -> Min/2  "<trqMotOperLim>"
  In2/1 -> Bus Selector1/1
  Bus Selector1/1 -> Min/3  "<trqMotnLim>"
  iDclnkLim/1 -> Bus Selector4/1
  TInvLim/1 -> Bus Selector3/1
  CANLim/1 -> Bus Selector2/1
  Bus Selector2/1 -> Min/4  "<trqMotCanLim>"
  Bus Selector3/1 -> Min/5  "<trqMotTInvLim>"
  Bus Selector4/1 -> Min/6  "<pwrMotUdclnkLim>"
  Gain/1 -> Max/1
  Bus Selector/2 -> Max/2  "<trqGenOperLim>"
  Bus Selector1/2 -> Max/3  "<trqGennLim>"
  Bus Selector2/2 -> Max/4  "<trqGenCanLim>"
  Bus Selector3/2 -> Max/5  "<trqGenTInvLim>"
  Bus Selector4/2 -> Max/6  "<signal1>"
  Min/1 -> Bus Creator/1  "trqMot"
  Max/1 -> Bus Creator/2  "trqMin"
  Bus Creator/1 -> Outport/1

== system TLC/TLC_TrqUdcLim ==
  note: uDcMin: Motor mode.
      | uDcMax: Generator mode.
      | Linear method
  udclink : Inport
  Bus Creator : BusCreator  Inputs=4
  Compare To Constant : simulink/Logic and Bit Operations/Compare To Constant  relop=<  const=1  OutDataTypeStr=boolean
  Compare To Constant1 : simulink/Logic and Bit Operations/Compare To Constant  relop=<  const=1  OutDataTypeStr=boolean
  GLB_PwrMax_P : Constant  Value=SC_PwrMax_P  OutDataTypeStr=single
  Gain : Gain  Gain=-1
  Product : Product
  Product1 : Product
  pwrGenUdclnkLim_T : Lookup_n-D  NumberOfTableDimensions=1  DataSpecification=Lookup table object  LookupTableObject=pwrGenUdclnkLim_T  BreakpointsForDimension1=[-8 -4 -2 0 5 6 7 8]  BeginIndexSearchUsingPreviousIndexResult=on  Table=[1 0.4 0.3 0 0 0 0 0]  ExtrapMethod=Clip  UseLastTableValue=on  InternalRulePriority=Speed  OutDataTypeStr=Inherit: Inherit from 'Table data'  RndMeth=Simplest
  pwrMotUdclnkLim_T : Lookup_n-D  NumberOfTableDimensions=1  DataSpecification=Lookup table object  LookupTableObject=pwrMotUdclnkLim_T  BreakpointsForDimension1=[-13 -11 -2 -1 0 1 2 5]  BeginIndexSearchUsingPreviousIndexResult=on  Table=[0 0 0 0.1 0.2 0.3 0.5 1]  ExtrapMethod=Clip  UseLastTableValue=on  InternalRulePriority=Speed  OutDataTypeStr=Inherit: Inherit from 'Table data'  RndMeth=Simplest  InputSameDT=off
  iDclnkLim : Outport  VectorParamsAs1DForOutWhenUnconnected=off
  wires:
  Compare To Constant1/1 -> Bus Creator/4  "bPwrMotUdclnkLimActv"
  Product1/1 -> Bus Creator/3  "pwrMotUdclnkLim"
  pwrMotUdclnkLim_T/1 -> Compare To Constant1/1, Product1/2
  Compare To Constant/1 -> Bus Creator/2  "bPwrGenUdclnkLimActv"
  Product/1 -> Gain/1  "pwrGenUdclnkLim"
  udclink/1 -> pwrMotUdclnkLim_T/1, pwrGenUdclnkLim_T/1
  pwrGenUdclnkLim_T/1 -> Compare To Constant/1, Product/2
  GLB_PwrMax_P/1 -> Product1/1, Product/1
  Bus Creator/1 -> iDclnkLim/1
  Gain/1 -> Bus Creator/1

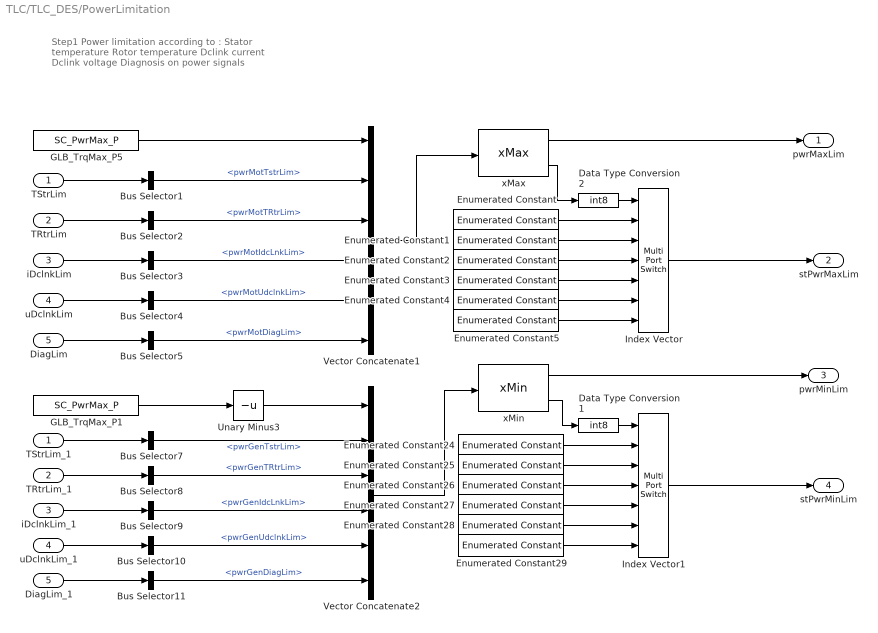
== system TLC/TLC_DES/PowerLimitation ==
  note: Step1 Power limitation according to :
      | Stator temperature
      | Rotor temperature
      | Dclink current
      | Dclink voltage
      | Diagnosis on power signals
  TStrLim : Inport
  TRtrLim : Inport  Port=2
  iDclnkLim : Inport  Port=3
  uDclnkLim : Inport  Port=4
  DiagLim : Inport  Port=5
  Bus Selector1 : BusSelector  OutputSignals=pwrMotTstrLim
  Bus Selector10 : BusSelector  OutputSignals=pwrGenUdclnkLim
  Bus Selector11 : BusSelector  OutputSignals=pwrGenDiagLim
  Bus Selector2 : BusSelector  OutputSignals=pwrMotTRtrLim
  Bus Selector3 : BusSelector  OutputSignals=pwrMotIdcLnkLim
  Bus Selector4 : BusSelector  OutputSignals=pwrMotUdclnkLim
  Bus Selector5 : BusSelector  OutputSignals=pwrMotDiagLim
  Bus Selector7 : BusSelector  OutputSignals=pwrGenTstrLim
  Bus Selector8 : BusSelector  OutputSignals=pwrGenTRtrLim
  Bus Selector9 : BusSelector  OutputSignals=pwrGenIdcLnkLim
  Data Type Conversion1 : DataTypeConversion  OutDataTypeStr=int8  SaturateOnIntegerOverflow=off  RndMeth=Floor
  Data Type Conversion2 : DataTypeConversion  OutDataTypeStr=int8  SaturateOnIntegerOverflow=off  RndMeth=Floor
  DiagLim_1 : InportShadow  Port=5
  Enumerated Constant : simulink/Sources/Enumerated Constant  OutDataTypeStr=Enum: TQL  Value=TQL.Inactive  SampleTime=inf
  Enumerated Constant1 : simulink/Sources/Enumerated Constant  OutDataTypeStr=Enum: TQL  Value=TQL.TStrMax  SampleTime=inf
  Enumerated Constant2 : simulink/Sources/Enumerated Constant  OutDataTypeStr=Enum: TQL  Value=TQL.TRtrMax  SampleTime=inf
  Enumerated Constant24 : simulink/Sources/Enumerated Constant  OutDataTypeStr=Enum: TQL  Value=TQL.Inactive  SampleTime=inf
  Enumerated Constant25 : simulink/Sources/Enumerated Constant  OutDataTypeStr=Enum: TQL  Value=TQL.TStrMax  SampleTime=inf
  Enumerated Constant26 : simulink/Sources/Enumerated Constant  OutDataTypeStr=Enum: TQL  Value=TQL.TRtrMax  SampleTime=inf
  Enumerated Constant27 : simulink/Sources/Enumerated Constant  OutDataTypeStr=Enum: TQL  Value=TQL.IdcMin  SampleTime=inf
  Enumerated Constant28 : simulink/Sources/Enumerated Constant  OutDataTypeStr=Enum: TQL  Value=TQL.UdcMax  SampleTime=inf
  Enumerated Constant29 : simulink/Sources/Enumerated Constant  OutDataTypeStr=Enum: TQL  Value=TQL.DIAPwrMin  SampleTime=inf
  Enumerated Constant3 : simulink/Sources/Enumerated Constant  OutDataTypeStr=Enum: TQL  Value=TQL.IdcMax  SampleTime=inf
  Enumerated Constant4 : simulink/Sources/Enumerated Constant  OutDataTypeStr=Enum: TQL  Value=TQL.UdcMin  SampleTime=inf
  Enumerated Constant5 : simulink/Sources/Enumerated Constant  OutDataTypeStr=Enum: TQL  Value=TQL.DIAPwrMax  SampleTime=inf
  GLB_TrqMax_P1 : Constant  Value=SC_PwrMax_P  OutDataTypeStr=single
  GLB_TrqMax_P5 : Constant  Value=SC_PwrMax_P  OutDataTypeStr=single
  Index Vector : MultiPortSwitch  Inputs=6  SaturateOnIntegerOverflow=off  InputSameDT=off
  Index Vector1 : MultiPortSwitch  Inputs=6  SaturateOnIntegerOverflow=off  InputSameDT=off
  TRtrLim_1 : InportShadow  Port=2
  TStrLim_1 : InportShadow
  Unary Minus3 : UnaryMinus
  Vector Concatenate1 : Concatenate  NumInputs=6
  Vector Concatenate2 : Concatenate  NumInputs=6
  iDclnkLim_1 : InportShadow  Port=3
  uDclnkLim_1 : InportShadow  Port=4
  xMax : MathLib/xMax  SystemSampleTime=-1  VariantActivationTime=update diagram  Latency=0  AutoFrameSizeCalculation=off
  xMin : MathLib/xMin  SystemSampleTime=-1  VariantActivationTime=update diagram  Latency=0  AutoFrameSizeCalculation=off
  pwrMaxLim : Outport  VectorParamsAs1DForOutWhenUnconnected=off
  stPwrMaxLim : Outport  Port=2  VectorParamsAs1DForOutWhenUnconnected=off
  pwrMinLim : Outport  Port=3  VectorParamsAs1DForOutWhenUnconnected=off
  stPwrMinLim : Outport  Port=4  VectorParamsAs1DForOutWhenUnconnected=off
  wires:
  TStrLim/1 -> Bus Selector1/1
  Bus Selector1/1 -> Vector Concatenate1/2  "<pwrMotTstrLim>"
  GLB_TrqMax_P5/1 -> Vector Concatenate1/1
  TRtrLim/1 -> Bus Selector2/1
  iDclnkLim/1 -> Bus Selector3/1
  uDclnkLim/1 -> Bus Selector4/1
  DiagLim/1 -> Bus Selector5/1
  xMax/1 -> pwrMaxLim/1
  TStrLim_1/1 -> Bus Selector7/1
  GLB_TrqMax_P1/1 -> Unary Minus3/1
  TRtrLim_1/1 -> Bus Selector8/1
  iDclnkLim_1/1 -> Bus Selector9/1
  uDclnkLim_1/1 -> Bus Selector10/1
  DiagLim_1/1 -> Bus Selector11/1
  Bus Selector2/1 -> Vector Concatenate1/3  "<pwrMotTRtrLim>"
  Bus Selector3/1 -> Vector Concatenate1/4  "<pwrMotIdcLnkLim>"
  Bus Selector4/1 -> Vector Concatenate1/5  "<pwrMotUdclnkLim>"
  Bus Selector5/1 -> Vector Concatenate1/6  "<pwrMotDiagLim>"
  Vector Concatenate1/1 -> xMax/1
  xMax/2 -> Data Type Conversion2/1
  Enumerated Constant/1 -> Index Vector/2
  Enumerated Constant1/1 -> Index Vector/3
  Enumerated Constant2/1 -> Index Vector/4
  Enumerated Constant3/1 -> Index Vector/5
  Enumerated Constant4/1 -> Index Vector/6
  Enumerated Constant5/1 -> Index Vector/7
  Unary Minus3/1 -> Vector Concatenate2/1
  Vector Concatenate2/1 -> xMin/1
  xMin/2 -> Data Type Conversion1/1
  Enumerated Constant24/1 -> Index Vector1/2
  Enumerated Constant25/1 -> Index Vector1/3
  Enumerated Constant26/1 -> Index Vector1/4
  Enumerated Constant27/1 -> Index Vector1/5
  Enumerated Constant28/1 -> Index Vector1/6
  Enumerated Constant29/1 -> Index Vector1/7
  Bus Selector8/1 -> Vector Concatenate2/3  "<pwrGenTRtrLim>"
  Bus Selector9/1 -> Vector Concatenate2/4  "<pwrGenIdcLnkLim>"
  Bus Selector10/1 -> Vector Concatenate2/5  "<pwrGenUdclnkLim>"
  Bus Selector7/1 -> Vector Concatenate2/2  "<pwrGenTstrLim>"
  Bus Selector11/1 -> Vector Concatenate2/6  "<pwrGenDiagLim>"
  xMin/1 -> pwrMinLim/1
  Data Type Conversion1/1 -> Index Vector1/1
  Data Type Conversion2/1 -> Index Vector/1
  Index Vector/1 -> stPwrMaxLim/1
  Index Vector1/1 -> stPwrMinLim/1

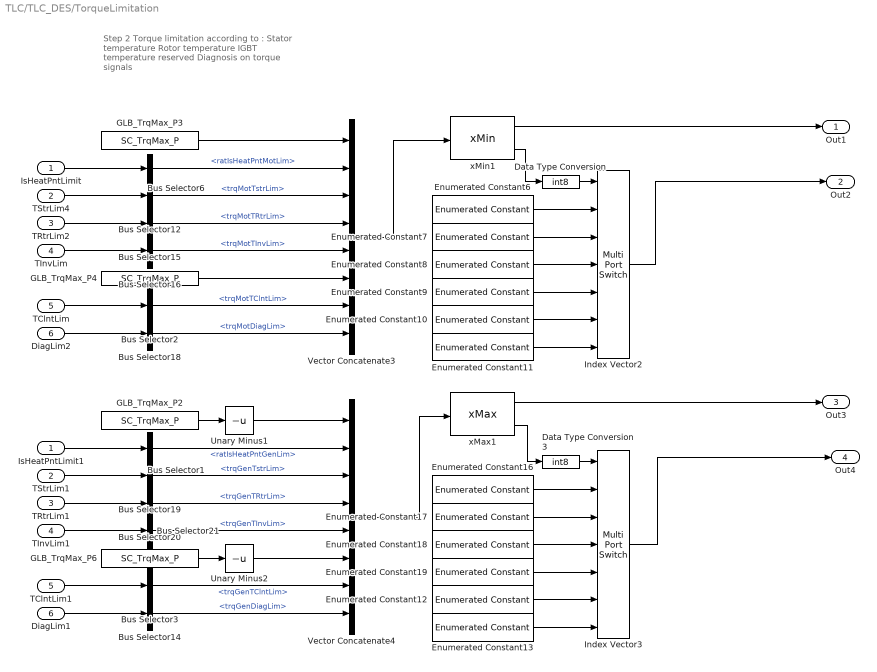
== system TLC/TLC_DES/TorqueLimitation ==
  note: Step 2 Torque limitation according to :
      | Stator temperature
      | Rotor temperature
      | IGBT temperature
      | reserved
      | Diagnosis on torque signals
  IsHeatPntLimit : Inport
  TStrLim4 : Inport  Port=2
  TRtrLim2 : Inport  Port=3
  TInvLim : Inport  Port=4
  TClntLim : Inport  Port=5
  DiagLim2 : Inport  Port=6
  Bus Selector1 : BusSelector  OutputSignals=ratIsHeatPntGenLim
  Bus Selector12 : BusSelector  OutputSignals=trqMotTstrLim
  Bus Selector14 : BusSelector  OutputSignals=trqGenDiagLim
  Bus Selector15 : BusSelector  OutputSignals=trqMotTRtrLim
  Bus Selector16 : BusSelector  OutputSignals=trqMotTInvLim
  Bus Selector18 : BusSelector  OutputSignals=trqMotDiagLim
  Bus Selector19 : BusSelector  OutputSignals=trqGenTstrLim
  Bus Selector2 : BusSelector  OutputSignals=trqMotTClntLim
  Bus Selector20 : BusSelector  OutputSignals=trqGenTRtrLim
  Bus Selector21 : BusSelector  OutputSignals=trqGenTInvLim
  Bus Selector3 : BusSelector  OutputSignals=trqGenTClntLim
  Bus Selector6 : BusSelector  OutputSignals=ratIsHeatPntMotLim
  Data Type Conversion : DataTypeConversion  OutDataTypeStr=int8  SaturateOnIntegerOverflow=off  RndMeth=Floor
  Data Type Conversion3 : DataTypeConversion  OutDataTypeStr=int8  SaturateOnIntegerOverflow=off  RndMeth=Floor
  DiagLim1 : InportShadow  Port=6
  Enumerated Constant{6,10,12,16} (4 alike) : simulink/Sources/Enumerated Constant  OutDataTypeStr=Enum: TQL  Value=TQL.Inactive  SampleTime=inf
  Enumerated Constant11 : simulink/Sources/Enumerated Constant  OutDataTypeStr=Enum: TQL  Value=TQL.DIATrqMax  SampleTime=inf
  Enumerated Constant13 : simulink/Sources/Enumerated Constant  OutDataTypeStr=Enum: TQL  Value=TQL.DIATrqMin  SampleTime=inf
  Enumerated Constant17 : simulink/Sources/Enumerated Constant  OutDataTypeStr=Enum: TQL  Value=TQL.TStrMax  SampleTime=inf
  Enumerated Constant18 : simulink/Sources/Enumerated Constant  OutDataTypeStr=Enum: TQL  Value=TQL.TRtrMax  SampleTime=inf
  Enumerated Constant19 : simulink/Sources/Enumerated Constant  OutDataTypeStr=Enum: TQL  Value=TQL.TIGBTMAX  SampleTime=inf
  Enumerated Constant7 : simulink/Sources/Enumerated Constant  OutDataTypeStr=Enum: TQL  Value=TQL.TStrMax  SampleTime=inf
  Enumerated Constant8 : simulink/Sources/Enumerated Constant  OutDataTypeStr=Enum: TQL  Value=TQL.TRtrMax  SampleTime=inf
  Enumerated Constant9 : simulink/Sources/Enumerated Constant  OutDataTypeStr=Enum: TQL  Value=TQL.TIGBTMAX  SampleTime=inf
  GLB_TrqMax_P{2..4,6} (4 alike) : Constant  Value=SC_TrqMax_P  OutDataTypeStr=single
  Index Vector2 : MultiPortSwitch  Inputs=6  SaturateOnIntegerOverflow=off  InputSameDT=off
  Index Vector3 : MultiPortSwitch  Inputs=6  SaturateOnIntegerOverflow=off  InputSameDT=off
  IsHeatPntLimit1 : InportShadow
  TClntLim1 : InportShadow  Port=5
  TInvLim1 : InportShadow  Port=4
  TRtrLim1 : InportShadow  Port=3
  TStrLim1 : InportShadow  Port=2
  Unary Minus1 : UnaryMinus
  Unary Minus2 : UnaryMinus
  Vector Concatenate3 : Concatenate  NumInputs=8
  Vector Concatenate4 : Concatenate  NumInputs=8
  xMax1 : MathLib/xMax  SystemSampleTime=-1  VariantActivationTime=update diagram  Latency=0  AutoFrameSizeCalculation=off
  xMin1 : MathLib/xMin  SystemSampleTime=-1  VariantActivationTime=update diagram  Latency=0  AutoFrameSizeCalculation=off
  Out1 : Outport  VectorParamsAs1DForOutWhenUnconnected=off
  Out2 : Outport  Port=2  VectorParamsAs1DForOutWhenUnconnected=off
  Out3 : Outport  Port=3  VectorParamsAs1DForOutWhenUnconnected=off
  Out4 : Outport  Port=4  VectorParamsAs1DForOutWhenUnconnected=off
  wires:
  TStrLim4/1 -> Bus Selector12/1
  TRtrLim2/1 -> Bus Selector15/1
  TInvLim/1 -> Bus Selector16/1
  DiagLim2/1 -> Bus Selector18/1
  TStrLim1/1 -> Bus Selector19/1
  GLB_TrqMax_P2/1 -> Unary Minus1/1
  TRtrLim1/1 -> Bus Selector20/1
  TInvLim1/1 -> Bus Selector21/1
  GLB_TrqMax_P6/1 -> Unary Minus2/1
  DiagLim1/1 -> Bus Selector14/1
  Vector Concatenate3/1 -> xMin1/1
  xMin1/2 -> Data Type Conversion/1
  Enumerated Constant6/1 -> Index Vector2/2
  Enumerated Constant7/1 -> Index Vector2/3
  Enumerated Constant8/1 -> Index Vector2/4
  Enumerated Constant9/1 -> Index Vector2/5
  Enumerated Constant10/1 -> Index Vector2/6
  Enumerated Constant11/1 -> Index Vector2/7
  GLB_TrqMax_P3/1 -> Vector Concatenate3/1
  GLB_TrqMax_P4/1 -> Vector Concatenate3/6
  Bus Selector12/1 -> Vector Concatenate3/3  "<trqMotTstrLim>"
  Bus Selector15/1 -> Vector Concatenate3/4  "<trqMotTRtrLim>"
  Bus Selector16/1 -> Vector Concatenate3/5  "<trqMotTInvLim>"
  Bus Selector18/1 -> Vector Concatenate3/8  "<trqMotDiagLim>"
  Vector Concatenate4/1 -> xMax1/1
  xMax1/2 -> Data Type Conversion3/1
  Enumerated Constant16/1 -> Index Vector3/2
  Enumerated Constant17/1 -> Index Vector3/3
  Enumerated Constant18/1 -> Index Vector3/4
  Enumerated Constant19/1 -> Index Vector3/5
  Enumerated Constant12/1 -> Index Vector3/6
  Enumerated Constant13/1 -> Index Vector3/7
  Unary Minus1/1 -> Vector Concatenate4/1
  Unary Minus2/1 -> Vector Concatenate4/6
  Bus Selector21/1 -> Vector Concatenate4/5  "<trqGenTInvLim>"
  Bus Selector14/1 -> Vector Concatenate4/8  "<trqGenDiagLim>"
  Bus Selector20/1 -> Vector Concatenate4/4  "<trqGenTRtrLim>"
  Bus Selector19/1 -> Vector Concatenate4/3  "<trqGenTstrLim>"
  xMin1/1 -> Out1/1
  Index Vector2/1 -> Out2/1
  xMax1/1 -> Out3/1
  Index Vector3/1 -> Out4/1
  Data Type Conversion/1 -> Index Vector2/1
  Data Type Conversion3/1 -> Index Vector3/1
  IsHeatPntLimit1/1 -> Bus Selector1/1
  Bus Selector1/1 -> Vector Concatenate4/2  "<ratIsHeatPntGenLim>"
  IsHeatPntLimit/1 -> Bus Selector6/1
  Bus Selector6/1 -> Vector Concatenate3/2  "<ratIsHeatPntMotLim>"
  TClntLim/1 -> Bus Selector2/1
  Bus Selector2/1 -> Vector Concatenate3/7  "<trqMotTClntLim>"
  TClntLim1/1 -> Bus Selector3/1
  Bus Selector3/1 -> Vector Concatenate4/7  "<trqGenTClntLim>"

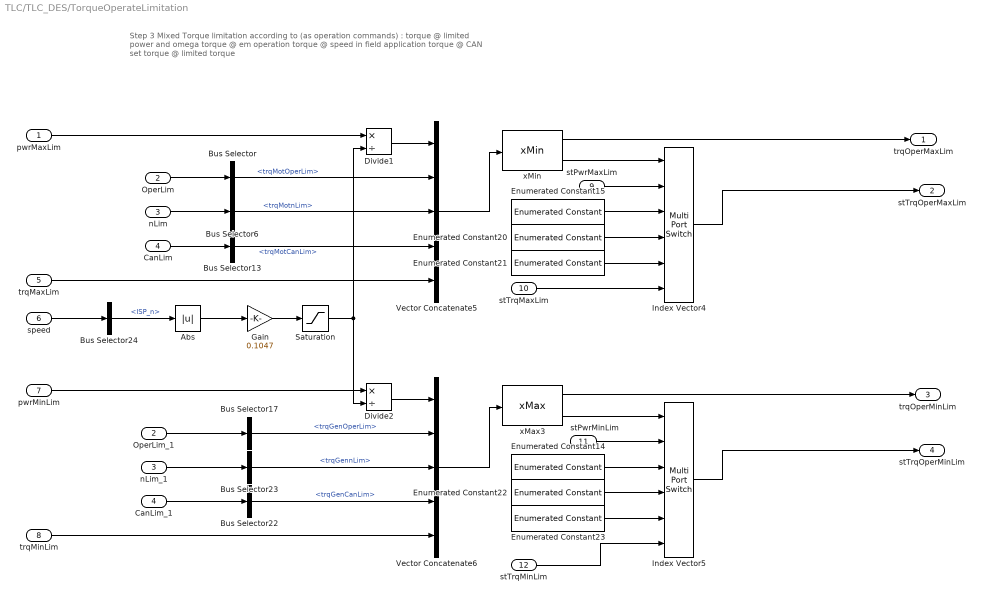
== system TLC/TLC_DES/TorqueOperateLimitation ==
  note: Step 3 Mixed Torque limitation according to (as operation commands) :
      | torque @ limited power and omega
      | torque @ em operation
      | torque @ speed in field application
      | torque @ CAN set
      | torque @ limited torque
  pwrMaxLim : Inport
  OperLim : Inport  Port=2
  nLim : Inport  Port=3
  CanLim : Inport  Port=4
  trqMaxLim : Inport  Port=5
  speed : Inport  Port=6
  pwrMinLim : Inport  Port=7
  trqMinLim : Inport  Port=8
  stPwrMaxLim : Inport  Port=9
  stTrqMaxLim : Inport  Port=10
  stPwrMinLim : Inport  Port=11
  stTrqMinLim : Inport  Port=12
  Abs : Abs  SaturateOnIntegerOverflow=off
  Bus Selector : BusSelector  OutputSignals=trqMotOperLim
  Bus Selector13 : BusSelector  OutputSignals=trqMotCanLim
  Bus Selector17 : BusSelector  OutputSignals=trqGenOperLim
  Bus Selector22 : BusSelector  OutputSignals=trqGenCanLim
  Bus Selector23 : BusSelector  OutputSignals=trqGennLim
  Bus Selector24 : BusSelector  OutputSignals=ISP_n
  Bus Selector6 : BusSelector  OutputSignals=trqMotnLim
  CanLim_1 : InportShadow  Port=4
  Divide1 : Product  Inputs=*/
  Divide2 : Product  Inputs=*/
  Enumerated Constant14 : simulink/Sources/Enumerated Constant  OutDataTypeStr=Enum: TQL  Value=TQL.OpRngElmGen  SampleTime=inf
  Enumerated Constant15 : simulink/Sources/Enumerated Constant  OutDataTypeStr=Enum: TQL  Value=TQL.OpRngElmMot  SampleTime=inf
  Enumerated Constant20 : simulink/Sources/Enumerated Constant  OutDataTypeStr=Enum: TQL  Value=TQL.nLim  SampleTime=inf
  Enumerated Constant21 : simulink/Sources/Enumerated Constant  OutDataTypeStr=Enum: TQL  Value=TQL.CANMax  SampleTime=inf
  Enumerated Constant22 : simulink/Sources/Enumerated Constant  OutDataTypeStr=Enum: TQL  Value=TQL.nLim  SampleTime=inf
  Enumerated Constant23 : simulink/Sources/Enumerated Constant  OutDataTypeStr=Enum: TQL  Value=TQL.CANMin  SampleTime=inf
  Gain : Gain  Gain=0.1047
  Index Vector4 : MultiPortSwitch  Inputs=5  SaturateOnIntegerOverflow=off  InputSameDT=off
  Index Vector5 : MultiPortSwitch  Inputs=5  SaturateOnIntegerOverflow=off  InputSameDT=off
  OperLim_1 : InportShadow  Port=2
  Saturation : Saturate  UpperLimit=inf  LowerLimit=300
  Vector Concatenate5 : Concatenate  NumInputs=5
  Vector Concatenate6 : Concatenate  NumInputs=5
  nLim_1 : InportShadow  Port=3
  xMax3 : MathLib/xMax  SystemSampleTime=-1  VariantActivationTime=update diagram  Latency=0  AutoFrameSizeCalculation=off
  xMin : MathLib/xMin  SystemSampleTime=-1  VariantActivationTime=update diagram  Latency=0  AutoFrameSizeCalculation=off
  trqOperMaxLim : Outport  VectorParamsAs1DForOutWhenUnconnected=off
  stTrqOperMaxLim : Outport  Port=2  VectorParamsAs1DForOutWhenUnconnected=off
  trqOperMinLim : Outport  Port=3  VectorParamsAs1DForOutWhenUnconnected=off
  stTrqOperMinLim : Outport  Port=4  VectorParamsAs1DForOutWhenUnconnected=off
  wires:
  OperLim/1 -> Bus Selector/1
  speed/1 -> Bus Selector24/1
  Abs/1 -> Gain/1
  Saturation/1 -> Divide1/2, Divide2/2
  Divide1/1 -> Vector Concatenate5/1
  Vector Concatenate5/1 -> xMin/1
  Bus Selector/1 -> Vector Concatenate5/2  "<trqMotOperLim>"
  nLim/1 -> Bus Selector6/1
  Bus Selector6/1 -> Vector Concatenate5/3  "<trqMotnLim>"
  CanLim/1 -> Bus Selector13/1
  Bus Selector13/1 -> Vector Concatenate5/4  "<trqMotCanLim>"
  Index Vector4/1 -> stTrqOperMaxLim/1
  xMin/2 -> Index Vector4/1
  Enumerated Constant15/1 -> Index Vector4/3
  Enumerated Constant20/1 -> Index Vector4/4
  Enumerated Constant21/1 -> Index Vector4/5
  OperLim_1/1 -> Bus Selector17/1
  Divide2/1 -> Vector Concatenate6/1
  Vector Concatenate6/1 -> xMax3/1
  Bus Selector17/1 -> Vector Concatenate6/2  "<trqGenOperLim>"
  nLim_1/1 -> Bus Selector23/1
  Bus Selector23/1 -> Vector Concatenate6/3  "<trqGennLim>"
  CanLim_1/1 -> Bus Selector22/1
  Bus Selector22/1 -> Vector Concatenate6/4  "<trqGenCanLim>"
  Index Vector5/1 -> stTrqOperMinLim/1
  xMax3/2 -> Index Vector5/1
  Enumerated Constant14/1 -> Index Vector5/3
  Enumerated Constant22/1 -> Index Vector5/4
  Enumerated Constant23/1 -> Index Vector5/5
  xMin/1 -> trqOperMaxLim/1
  xMax3/1 -> trqOperMinLim/1
  pwrMaxLim/1 -> Divide1/1
  pwrMinLim/1 -> Divide2/1
  trqMaxLim/1 -> Vector Concatenate5/5
  trqMinLim/1 -> Vector Concatenate6/5
  Bus Selector24/1 -> Abs/1  "<ISP_n>"
  stTrqMinLim/1 -> Index Vector5/6
  stPwrMaxLim/1 -> Index Vector4/2
  stTrqMaxLim/1 -> Index Vector4/6
  stPwrMinLim/1 -> Index Vector5/2
  Gain/1 -> Saturation/1

== system TLC/TLC_EM/CANLim ==
  note: Maximum/Minimum from CAN:
      | ISC_TrqEMMax
      | ISC_TrqEMMin
  In1 : Inport
  In2 : Inport  Port=2
  Bus Creator : BusCreator  Inputs=2
  CANLim : Outport  VectorParamsAs1DForOutWhenUnconnected=off
  wires:
  In1/1 -> Bus Creator/1  "trqMotCanLim"
  In2/1 -> Bus Creator/2  "trqGenCanLim"
  Bus Creator/1 -> CANLim/1

== system TLC/TLC_EM/DiafLim ==
  note: Not realized as the diagnosis implemetation not clear.
      | 4-level Function planned:
      | Diagnosis level 1: scale_P = 0
      | Diagnosis level 2: scale_P = 0.25
      | Diagnosis level 3: scale_P = 0.33
      | Diagnosis level 4: scale_P = 0.5
  Bus Creator : BusCreator  Inputs=8
  Constant{,1..3} (4 alike) : Constant  Value=0  OutDataTypeStr=boolean
  GLB_PwrMax_P : Constant  Value=SC_PwrMax_P  OutDataTypeStr=single
  GLB_PwrMax_P1 : Constant  Value=SC_TrqMax_P  OutDataTypeStr=single
  Signal Conversion : SignalConversion  OverrideOpt=off
  Signal Conversion1 : SignalConversion  OverrideOpt=off
  Unary Minus1 : UnaryMinus
  Unary Minus3 : UnaryMinus
  Out1 : Outport  VectorParamsAs1DForOutWhenUnconnected=off
  wires:
  GLB_PwrMax_P/1 -> Unary Minus3/1, Signal Conversion/1
  Bus Creator/1 -> Out1/1
  Unary Minus3/1 -> Bus Creator/2  "pwrGenDiagLim"
  Constant/1 -> Bus Creator/3  "bPwrMotDiagLimActv"
  Constant1/1 -> Bus Creator/4  "bPwrGenDiagLimActv"
  GLB_PwrMax_P1/1 -> Unary Minus1/1, Signal Conversion1/1
  Unary Minus1/1 -> Bus Creator/6  "trqGenDiagLim"
  Constant2/1 -> Bus Creator/8  "bTrqGenDiagLimActv"
  Constant3/1 -> Bus Creator/7  "bTrqMotDiagLimActv"
  Signal Conversion/1 -> Bus Creator/1  "pwrMotDiagLim"
  Signal Conversion1/1 -> Bus Creator/5  "trqMotDiagLim"
